simulink model "QPSK1"  (Simulink 10.1)
settings: Solver=VariableStepAuto  StartTime=0.0  StopTime=1000  RelTol=1e-3
undefined symbols (not defined in the file): j
libraries: dsp_blocks x7
settings Model: Creator=rayan  LastModifiedBy=rayan
settings DataIOCC: SaveFormat=Dataset  ReturnWorkspaceOutputs=on
settings OptimizationCC: LifeSpan=auto
settings DebuggingCC: UnderspecifiedInitializationDetection=Simplified  MergeDetectMultiDrivingBlocksExec=error  SFUnexpectedBacktrackingDiag=error  SFNoUnconditionalDefaultTransitionDiag=error  SFExecutionAtInitializationDiag=warning  ArithmeticOperatorsInVariantConditions=error
settings HardwareCC: ProdBitPerPointer=64  ProdBitPerSizeT=64  ProdBitPerPtrDiffT=64  ProdLargestAtomicFloat=Float  ProdIntDivRoundTo=Zero  ProdEndianess=LittleEndian  ProdWordSize=64  ProdHWDeviceType=Intel->x86-64 (Windows64)
settings ModelReferenceCC: PropagateSignalLabelsOutOfModel=on
settings SFSimCC: SimUseLocalCustomCode=on  CustomCodeUndefinedFunction=FilterOut
settings RTWCC: RTWUseLocalCustomCode=on
settings CodeAppCC: StateflowObjectComments=off
settings GRTTargetCC: TargetLangStandard=C99 (ISO)  CombineOutputUpdateFcns=on  GRTInterface=off
settings ConfigComp: CovMetricSettings=dwe  CovHtmlReporting=off  CovSaveCumulativeToWorkspaceVar=off  CovSaveSingleToWorkspaceVar=off  CovExternalEMLEnable=on

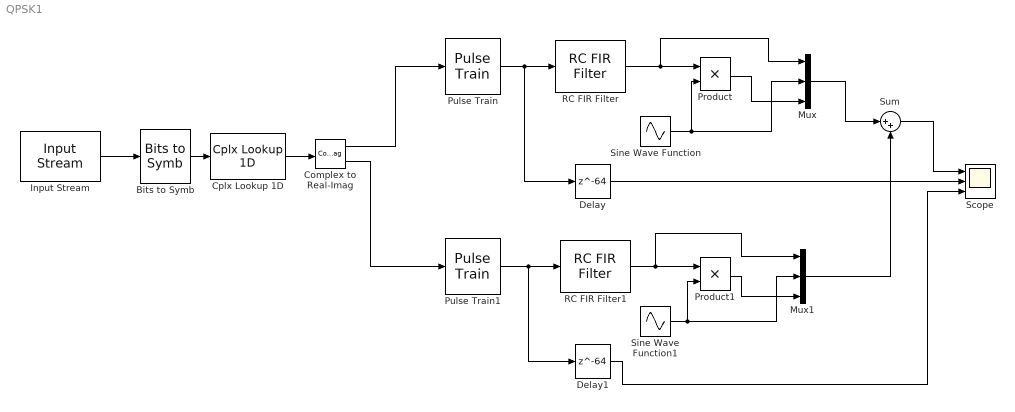
== system QPSK1 ==
  Bits to Symb : dsp_blocks/Conversions/Bits to Symb
  Complex to Real-Imag : ComplexToRealImag
  Cplx Lookup 1D : dsp_blocks/Conversions/Cplx Lookup 1D  table=[1 j -1 -j]
  Delay : Delay  DelayLength=64
  Delay1 : Delay  DelayLength=64
  Input Stream : dsp_blocks/Sources//Sinks/Input Stream  period=50  width=2  fname=rand.mat
  Mux : Mux  Inputs=3
  Mux1 : Mux  Inputs=3
  Product : Product
  Product1 : Product
  Pulse Train : dsp_blocks/Conversions/Pulse Train  period=50
  Pulse Train1 : dsp_blocks/Conversions/Pulse Train  period=50
  RC FIR Filter : dsp_blocks/Filters/RC FIR Filter  period=50  beta=0.5  root=off  filt_len=128  win_type=on
  RC FIR Filter1 : dsp_blocks/Filters/RC FIR Filter  period=50  beta=0.5  root=off  filt_len=128  win_type=on
  Scope : Scope  NumInputPorts=3
  Sine Wave Function : Sin  Frequency=2*pi*0.1  Phase=pi/2  SampleTime=0
  Sine Wave Function1 : Sin  Frequency=2*pi*0.1  SampleTime=0
  Sum : Sum  Inputs=|++
  wires:
  Input Stream/1 -> Bits to Symb/1
  Bits to Symb/1 -> Cplx Lookup 1D/1
  Pulse Train/1 -> Delay/1, RC FIR Filter/1
  Delay/1 -> Scope/2
  RC FIR Filter/1 -> Product/1, Mux/1
  Product/1 -> Mux/3
  Sine Wave Function/1 -> Mux/2, Product/2
  Cplx Lookup 1D/1 -> Complex to Real-Imag/1
  Complex to Real-Imag/1 -> Pulse Train/1
  Complex to Real-Imag/2 -> Pulse Train1/1
  Pulse Train1/1 -> Delay1/1, RC FIR Filter1/1
  RC FIR Filter1/1 -> Mux1/1, Product1/1
  Product1/1 -> Mux1/3
  Sine Wave Function1/1 -> Product1/2, Mux1/2
  Mux/1 -> Sum/1
  Mux1/1 -> Sum/2
  Sum/1 -> Scope/1
  Delay1/1 -> Scope/3
